simulink model "linear1"  (Simulink 6.2)
settings: Solver=ode45  StartTime=0.0  StopTime=0.1  RelTol=1e-3
libraries: simulink x2
settings Model: Creator=Alexander  ModifiedByFormat=Alexander  LastModifiedBy=Alexander
settings DebuggingCC: SolverPrmCheckMsg=warning

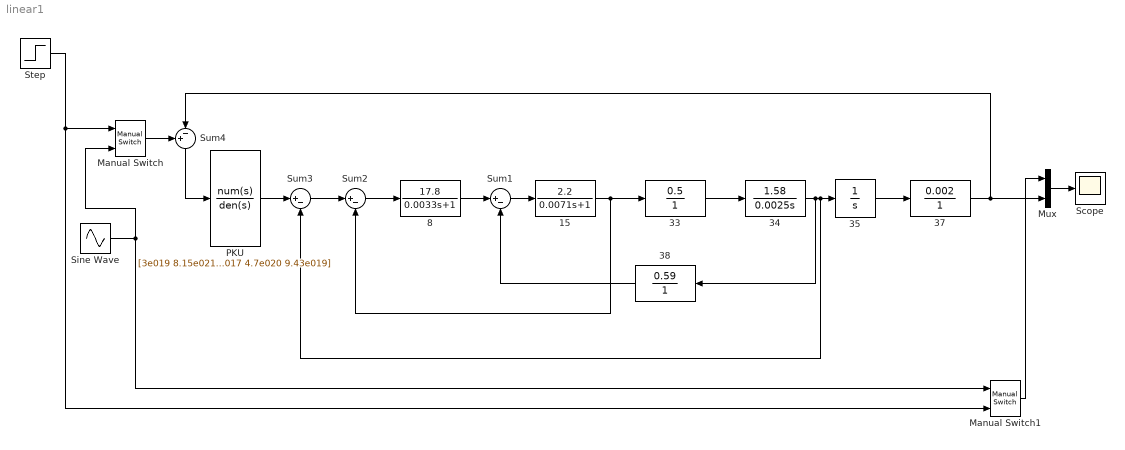
== system linear1 ==
  15 : TransferFcn  Numerator=[2.2]  Denominator=[0.0071 1]
  33 : TransferFcn  Numerator=[0.5]  Denominator=[1]
  34 : TransferFcn  Numerator=[1.58]  Denominator=[0.0025 0]
  35 : TransferFcn  Denominator=[1 0]
  37 : TransferFcn  Numerator=[0.002]  Denominator=[1]
  38 : TransferFcn  Orientation=left  Numerator=[0.59]  Denominator=[1]
  8 : TransferFcn  Numerator=[17.8]  Denominator=[0.0033 1]
  Manual Switch : simulink/Signal Routing/Manual Switch  sw=1  action=0
  Manual Switch1 : simulink/Signal Routing/Manual Switch  sw=0  action=0
  Mux : Mux  Inputs=2
  PKU : TransferFcn  Numerator=[3e019 8.15e021 4.4e024 1.5e026 0]  Denominator=[0.059 1.1e004 6.5e008 1.5e013 1.43e017 4.7e020 9.43e019]
  Scope : Scope
      settings: YMin=0  YMax=1.75e-006
  Sine Wave : Sin  Frequency=240  SampleTime=0
  Step : Step  Time=0  SampleTime=0
  Sum1 : Sum  Inputs=|+-
  Sum2 : Sum  Inputs=|+-
  Sum3 : Sum  Inputs=|+-
  Sum4 : Sum  Orientation=down  Inputs=+-|
  wires:
  34/1 -> 38/1, 35/1, Sum3/2
  38/1 -> Sum1/2
  8/1 -> Sum1/1
  Sum3/1 -> Sum2/1
  Sum2/1 -> 8/1
  Sum4/1 -> PKU/1
  37/1 -> Sum4/2, Mux/2
  Mux/1 -> Scope/1
  Manual Switch/1 -> Sum4/1
  Step/1 -> Manual Switch/1, Manual Switch1/2
  Sum1/1 -> 15/1
  15/1 -> 33/1, Sum2/2
  33/1 -> 34/1
  35/1 -> 37/1
  PKU/1 -> Sum3/1
  Manual Switch1/1 -> Mux/1
  Sine Wave/1 -> Manual Switch/2, Manual Switch1/1
